simulink model "Helmholtz_PF"  (Simulink 8.0)
settings: Solver=FixedStepDiscrete  StartTime=0.0  StopTime=1.0  FixedStep=1.0  RelTol=1e-3
libraries: Network_library x5
settings Model: Creator=mur  LastModifiedBy=mur
settings DataIOCC: SignalLoggingSaveFormat=ModelDataLogs
settings DebuggingCC: FcnCallInpInsideContextMsg=UseLocalSettings
settings GRTTargetCC: CombineOutputUpdateFcns=off  GRTInterface=on

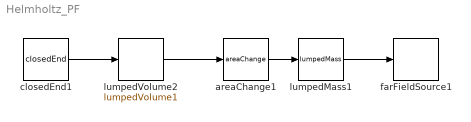
== system Helmholtz_PF ==
  areaChange1 : Network_library/areaChange  element=areaChange  aj=pi/4 * .05^2  D=0
      settings: AttributesFormatString=%<aj> m^2
  closedEnd1 : Network_library/closedEnd  element=closedEnd  loc=Upstream  c=340  Mach=0.  rho=1.2  D=0  a=1
  farFieldSource1 : Network_library/farFieldSource  element=farFieldSource  loc=Downstream  Amp=100  c=100  Mach=0.1  rho=1.2  D=1  a=1
      settings: AttributesFormatString=%<Amp> Pa
  lumpedMass1 : Network_library/lumpedMass  element=lumpedMass  Flag=Equivalent length  Leq=1e-2  Veq=1  meq=1e-3
      settings: AttributesFormatString=%<Leq> m
  lumpedVolume2 : Network_library/lumpedVolume1  element=lumpedVolume  Flag=Equivalent length  Leq=.5  Veq=1
      settings: AttributesFormatString=%<Leq> m
  wires:
  closedEnd1/1 -> lumpedVolume2/1
  lumpedVolume2/1 -> areaChange1/1
  areaChange1/1 -> lumpedMass1/1
  lumpedMass1/1 -> farFieldSource1/1
